simulink model "normalOperations_fsm"  (R2022a)
settings: Solver=VariableStepAuto  StartTime=0.0  StopTime=10.0  RelTol=1e-3
settings Model: Creator=Nate  LastModifiedBy=Nate
settings DebuggingCC: UnconnectedInputMsg=warning  UnconnectedOutputMsg=warning  UnconnectedLineMsg=warning
settings RTWCC: DLArmComputeVersion=19.05

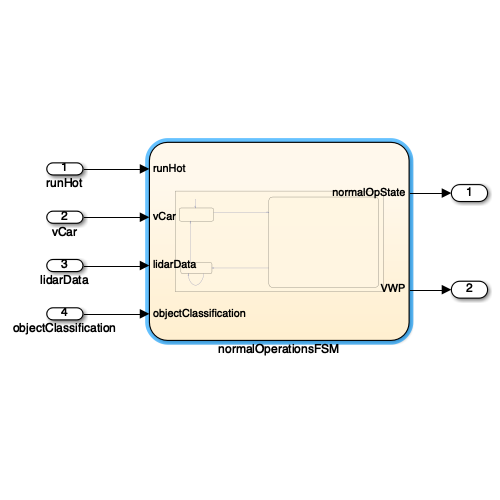
[thumbnail: Simulink's stored preview of the top-level diagram]
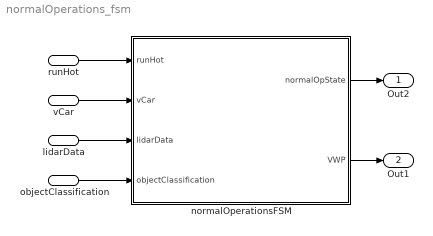
== system normalOperations_fsm ==
  runHot : Inport
  vCar : Inport  Port=2
  lidarData : Inport  Port=3
  objectClassification : Inport  Port=4
  normalOperationsFSM : Stateflow chart  TreatAsAtomicUnit=on
  Out2 : Outport
  Out1 : Outport  Port=2
  wires:
  runHot/1 -> normalOperationsFSM/1(runHot)
  vCar/1 -> normalOperationsFSM/2(vCar)
  lidarData/1 -> normalOperationsFSM/3(lidarData)
  objectClassification/1 -> normalOperationsFSM/4(objectClassification)
  normalOperationsFSM/1(normalOpState) -> Out2/1
  normalOperationsFSM/2(VWP) -> Out1/1

== stateflow chart normalOperations_fsm/normalOperationsFSM ==
  state normalOperations [group]
    state autonomous_mode
      en: normalOpState = 1
      du:
      updateObstaclesInProjectedOccupancyZones(ActiveObjectList, VWP, ...
      objectClassification, lidarData)
      du:
      curObject = sort(ActiveObjectList)
      du:
      SubMachineRunning = StopSignEnable || VariableStopEnable || ...
      LocalRerouteEnable || GlobalRerouteEnable
      if curObject == None
      disp("curObject is None")
      elseif  curObject == stopSign
      StopSignEnable = true
      VariableStopEnable = false
      LocalRerouteEnable = false
      GlobalRerouteEnable = false
      elseif curObject == stopLight || RR || movingObstacle
      StopSignEnable = false
      VariableStopEnable = true
      LocalRerouteEnable = false
      GlobalRerouteEnable = false
      elseif requiresLocalReroute(curObject)
      StopSignEnable = false
      VariableStopEnable = false
      LocalRerouteEnable = true
      GlobalRerouteEnable = false
      else
      StopSignEnable = false
      VariableStopEnable = false
      LocalRerouteEnable = false
      GlobalRerouteEnable = true
      end
      du:
      if SubMachineRunning == false && abs(vCar - LastSeenSpeedLimit) > 0.5
      SpeedChangeEnable = true
      end
    state manual_mode
      en: normalOpState = 0
      en: ActiveObjectList = []
    state wait_for_stopped
      en: normalOpState = 2
    (default) -> manual_mode
    manual_mode -> autonomous_mode : [runHot == true && VWP.length > 0]
    wait_for_stopped -> manual_mode [order 1] : [vCar == 0]
    autonomous_mode -> wait_for_stopped [order 1] : [VWP.length == 0]
        | {updateVWP(VWP, distance)}
    wait_for_stopped -> wait_for_stopped [order 2]
    autonomous_mode -> autonomous_mode [order 2] : {waypointHandshake()}
  data: distance constant double; runHot input; movingObstacle constant double; stopLight constant double; stopSign constant double; None constant double; vCar input; lidarData input; objectClassification input; SpeedChangeEnable data_store_memory; ReroutingEnable data_store_memory; curObject local; StopSignEnable data_store_memory; ActiveObjectList data_store_memory; VariableStopEnable data_store_memory; SubMachineRunning data_store_memory; RR constant double; normalOpState output; VWP output; LastSeenSpeedLimit data_store_memory; LocalRerouteEnable data_store_memory; GlobalRerouteEnable data_store_memory
